simulink model "robot_capteur_etu"  (R2021a)
settings: Solver=VariableStepAuto  StartTime=0.0  StopTime=10.0  RelTol=1e-3
values from neighbouring files (symbols this model uses):
  K = -place(A,B,poles)    [matrices.m]    (also in simu_robot_etu.m = [0.6700, 19.9055,1.0747,1.9614])
  ue = 0    [simu_robot_etu.m]
  x0 = [0 pi/10 0 0]    [simu_robot_etu.m]
  xe = [0 0 0 0]'    [simu_robot_etu.m]
settings Model: Creator=melyesse  LastModifiedBy=melyesse

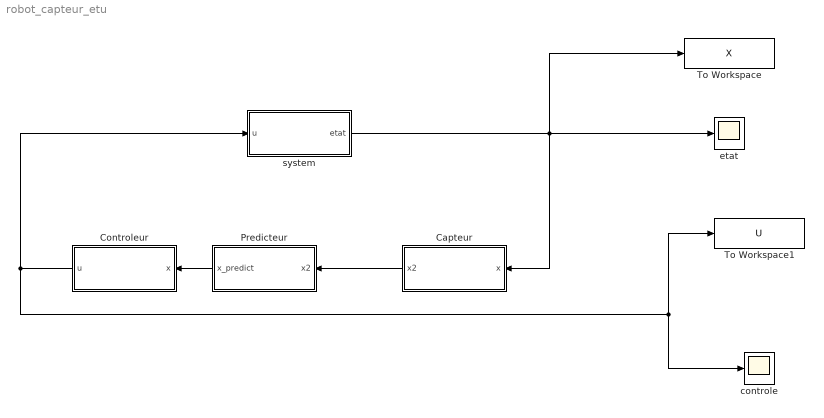
== system robot_capteur_etu ==
  Capteur : Subsystem
  Controleur : Subsystem
  Predicteur : Subsystem
  To Workspace : ToWorkspace  VariableName=X  SaveFormat=Timeseries  SampleTime=-1
  To Workspace1 : ToWorkspace  VariableName=U  SaveFormat=Timeseries  SampleTime=-1
  controle : Scope
  etat : Scope
  system : Subsystem
  wires:
  Capteur/1(x2) -> Predicteur/1(x2)
  system/1(etat) -> etat/1, To Workspace/1, Capteur/1(x)
  Predicteur/1(x_predict) -> Controleur/1(x)
  Controleur/1(u) -> system/1(u), controle/1, To Workspace1/1

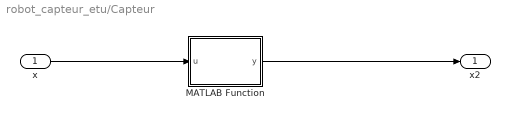
== system robot_capteur_etu/Capteur ==
  x : Inport
  MATLAB Function : MATLAB Function  TreatAsAtomicUnit=on
  x2 : Outport
  wires:
  x/1 -> MATLAB Function/1(u)
  MATLAB Function/1(y) -> x2/1

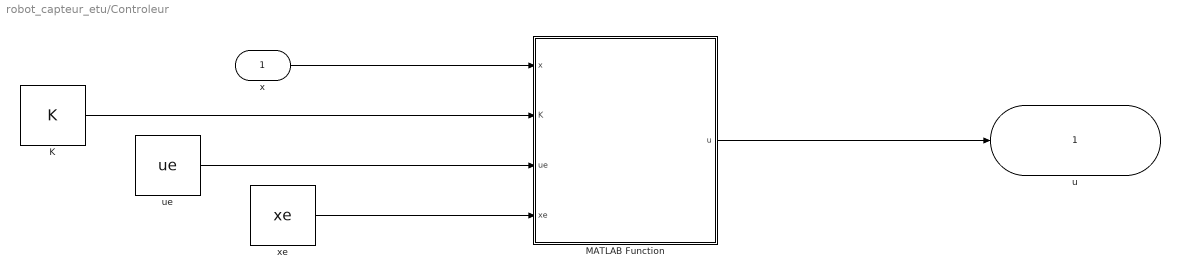
== system robot_capteur_etu/Controleur ==
  x : Inport
  K : Constant  Value=K  VectorParams1D=off
  MATLAB Function : MATLAB Function  TreatAsAtomicUnit=on
  ue : Constant  Value=ue
  xe : Constant  Value=xe
  u : Outport
  wires:
  xe/1 -> MATLAB Function/4(xe)
  ue/1 -> MATLAB Function/3(ue)
  x/1 -> MATLAB Function/1(x)
  MATLAB Function/1(u) -> u/1
  K/1 -> MATLAB Function/2(K)

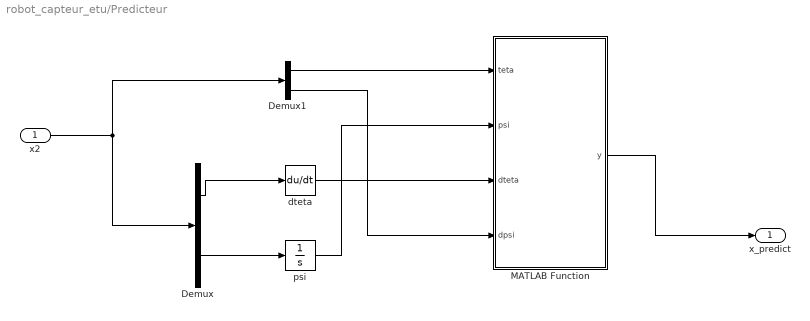
== system robot_capteur_etu/Predicteur ==
  x2 : Inport
  Demux : Demux  Outputs=2
  Demux1 : Demux  Outputs=2
  MATLAB Function : MATLAB Function  TreatAsAtomicUnit=on
  dteta : Derivative
  psi : Integrator
  x_predict : Outport
  wires:
  x2/1 -> Demux1/1, Demux/1
  Demux/1 -> dteta/1
  Demux/2 -> psi/1
  MATLAB Function/1(y) -> x_predict/1
  Demux1/1 -> MATLAB Function/1(teta)
  psi/1 -> MATLAB Function/2(psi)
  Demux1/2 -> MATLAB Function/4(dpsi)
  dteta/1 -> MATLAB Function/3(dteta)

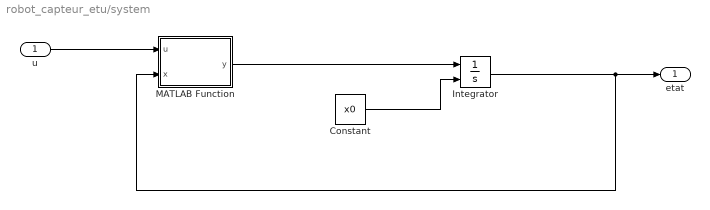
== system robot_capteur_etu/system ==
  u : Inport
  Constant : Constant  Value=x0
  Integrator : Integrator  InitialConditionSource=external
  MATLAB Function : MATLAB Function  TreatAsAtomicUnit=on
  etat : Outport
  wires:
  MATLAB Function/1(y) -> Integrator/1
  u/1 -> MATLAB Function/1(u)
  Constant/1 -> Integrator/2
  Integrator/1 -> MATLAB Function/2(x), etat/1

== matlab function robot_capteur_etu/Predicteur/MATLAB Function ==
  data: teta input; psi input; y output; dteta input; dpsi input
function y = fcn(teta,psi,dteta,dpsi)

y = [teta;dteta;psi;dpsi];

== matlab function robot_capteur_etu/system/MATLAB Function ==
  data: u input; y output; x input
function y = fcn(u,x)
y = fonction(x,u);

== matlab function robot_capteur_etu/Controleur/MATLAB Function ==
  data: x input; u output; K input; ue input; xe input
function u = fcn(x,K,ue,xe)
u = ue + (K*(x-xe));

== matlab function robot_capteur_etu/Capteur/MATLAB Function ==
  data: u input; y output
function y = fcn(u)

y = [u(1) ; u(4)];
